simulink library "TLMLib"  (Simulink 8.8)
settings: Solver=VariableStepAuto  StartTime=0.0  StopTime=10.0  RelTol=1e-3
libraries: mblibv1 x12, TLMLib x2
settings Model: Creator=Administrator  LastModifiedBy=robbr48  ExtModeAutoUpdateStatusClock=off

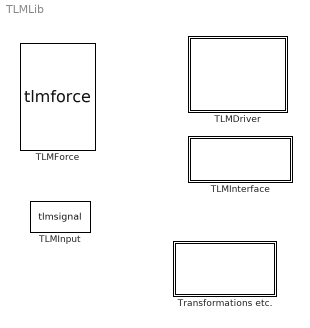
== system TLMLib ==
  TLMDriver : Subsystem
  TLMForce : S-Function  FunctionName=tlmforce  SFunctionDeploymentMode=off  EnableBusSupport=off  mask(TLMForceInterface){}
      mask help:
      | The TLM force interface enables Simulink to participate in TLM Co-Simulations.
      | The interface consists of communication port and a cartesian coordiante system.
      mask Help:
      | The input are:<br>
      | R = Three dimensional position vector, describing the interface location relative the inertial system.<br>
      | A = Orientation matrix 3x3 describing the interface orientation relative the inertial system.<br>
      | vR = Three dimensional velocity vector. <br>
      | Omega = Three dimensional vector describing the rotational velocity.<br>
      | <br>
      | The outputs are:<br>
      | F = Reaction force in the interface.<br>
      | M = Reaction moment in the interface.<br>
      mask Display:
      | port_label('input',1,'R');
      | port_label('input',2,'A');
      | port_label('output',3,'R');
      | port_label('output',4,'A');
      | color('red');
      | port_label('input',3,'vR');
      | port_label('input',4,'Omega');
      | port_label('output',1,'F');
      | port_label('output',2,'M');
  TLMInput : S-Function  FunctionName=tlmsignal  SFunctionDeploymentMode=off  EnableBusSupport=off
      mask Display:
      | port_label('input',1,'u1');
      | port_label('input',2,'u2');
      | color('red');
      | port_label('output',1,'y1');
      | port_label('output',2,'y2');
  TLMInterface : Subsystem
  Transformations etc. : Subsystem
      mask Display: disp('TOOLS')

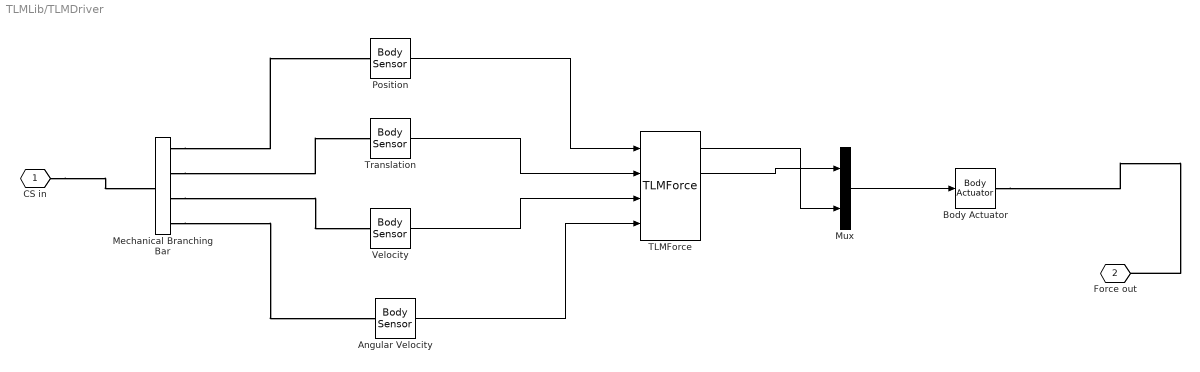
== system TLMLib/TLMDriver ==
  Angular Velocity : mblibv1/Sensors &  Actuators/Body Sensor  SystemSampleTime=-1  PhysicalDomain=Mechanical  PortType=blob  Muxed=on  Pose=off  Angle=on  AngleUnits=deg  ArcVelocity=on  ArcVelocityUnits=rad/s  ArcAcceleration=off  ArcAccelerationUnits=deg/s^2  CoordPosition=off  CoordPositionUnits=m  Velocity=off  VelocityUnits=m/s  Acceleration=off  AccelerationUnits=m/s^2  Quaternion=on  QuaternionDT=off  QuaternionDDT=off  QuaternionUnits=off  OutputVector=[1]  ActiveIO=off  Width=1  DialogClass=MechanicalSensorBlock  ReferenceFrame=Absolute (World)
  Body Actuator : mblibv1/Sensors &  Actuators/Body Actuator  SystemSampleTime=-1  PhysicalDomain=Mechanical  PortType=blob  ActuationStyle=Force  AngleUnits=deg  ArcVelocityUnits=deg/s  ArcAccelerationUnits=deg/s^2  CoordPositionUnits=m  VelocityUnits=m/s  AccelerationUnits=m/s^2  ForceUnits=N  TorqueUnits=N*m  ActiveIO=off  Width=1  DialogClass=MechanicalActuatorBlock  ReferenceFrame=Absolute (World)  Angle=off  CoordPosition=on  Force=on  Torque=on
  Mechanical Branching Bar : mblibv1/Utilities/Mechanical Branching Bar  PhysicalDomain=mechanical  SubClassName=Unknown  LeftPortType=blob  RightPortType=blob  LConnTagsString=_newl0  RConnTagsString=__newr0|SA2|SA3|SA4  DialogClass=MechanicalBranchingBarBlock  NumSAPorts=4
  Mux : Mux  Inputs=[3 3]
  Position : mblibv1/Sensors &  Actuators/Body Sensor  SystemSampleTime=-1  PhysicalDomain=Mechanical  PortType=blob  Muxed=on  Pose=off  Angle=on  AngleUnits=deg  ArcVelocity=off  ArcVelocityUnits=deg/s  ArcAcceleration=off  ArcAccelerationUnits=deg/s^2  CoordPosition=on  CoordPositionUnits=m  Velocity=off  VelocityUnits=m/s  Acceleration=off  AccelerationUnits=m/s^2  Quaternion=on  QuaternionDT=off  QuaternionDDT=off  QuaternionUnits=off  OutputVector=[1]  ActiveIO=off  Width=1  DialogClass=MechanicalSensorBlock  ReferenceFrame=Absolute (World)
  TLMForce : TLMLib/TLMForce
  Translation : mblibv1/Sensors &  Actuators/Body Sensor  SystemSampleTime=-1  PhysicalDomain=Mechanical  PortType=blob  Muxed=on  Pose=on  Angle=on  AngleUnits=deg  ArcVelocity=off  ArcVelocityUnits=deg/s  ArcAcceleration=off  ArcAccelerationUnits=deg/s^2  CoordPosition=off  CoordPositionUnits=m  Velocity=off  VelocityUnits=m/s  Acceleration=off  AccelerationUnits=m/s^2  Quaternion=on  QuaternionDT=off  QuaternionDDT=off  QuaternionUnits=off  OutputVector=[1]  ActiveIO=off  Width=1  DialogClass=MechanicalSensorBlock  ReferenceFrame=Absolute (World)
  Velocity : mblibv1/Sensors &  Actuators/Body Sensor  SystemSampleTime=-1  PhysicalDomain=Mechanical  PortType=blob  Muxed=on  Pose=off  Angle=on  AngleUnits=deg  ArcVelocity=off  ArcVelocityUnits=deg/s  ArcAcceleration=off  ArcAccelerationUnits=deg/s^2  CoordPosition=off  CoordPositionUnits=m  Velocity=on  VelocityUnits=m/s  Acceleration=off  AccelerationUnits=m/s^2  Quaternion=on  QuaternionDT=off  QuaternionDDT=off  QuaternionUnits=off  OutputVector=[1]  ActiveIO=off  Width=1  DialogClass=MechanicalSensorBlock  ReferenceFrame=Absolute (World)
  CS in : PMIOPort  Tag=PMCPort  Port=1  Side=Left
  Force out : PMIOPort  Tag=PMCPort  Port=2  Side=Right
  wires:
  Mux/1 -> Body Actuator/1
  TLMForce/1 -> Mux/2
  TLMForce/2 -> Mux/1
  Angular Velocity/1 -> TLMForce/4
  Velocity/1 -> TLMForce/3
  Translation/1 -> TLMForce/2
  Position/1 -> TLMForce/1
  connections:
  Mechanical Branching Bar/RConn3 -- Velocity/LConn1
  Mechanical Branching Bar/RConn2 -- Translation/LConn1
  Body Actuator/RConn1 -- Force out/RConn1
  CS in/RConn1 -- Mechanical Branching Bar/LConn1
  Mechanical Branching Bar/RConn4 -- Angular Velocity/LConn1
  Mechanical Branching Bar/RConn1 -- Position/LConn1

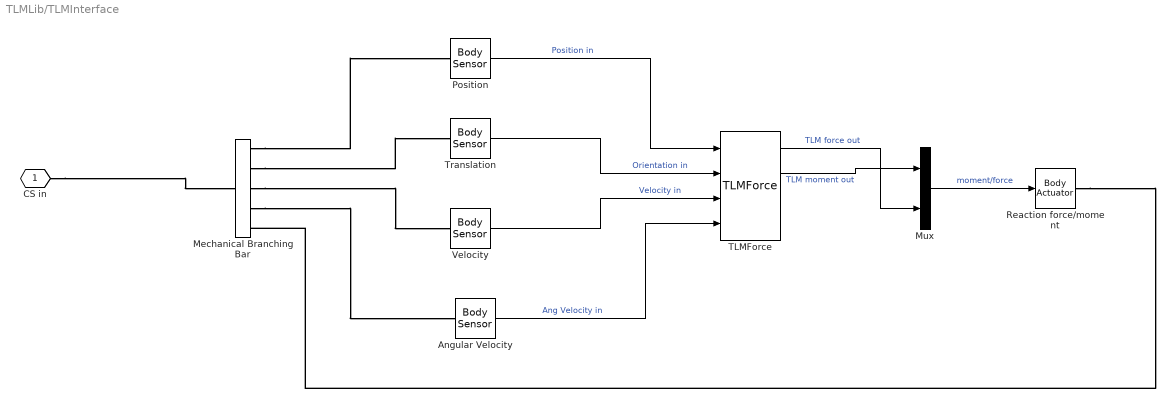
== system TLMLib/TLMInterface ==
  Angular Velocity : mblibv1/Sensors &  Actuators/Body Sensor  SystemSampleTime=-1  PhysicalDomain=Mechanical  PortType=blob  Muxed=on  Pose=off  Angle=on  AngleUnits=deg  ArcVelocity=on  ArcVelocityUnits=rad/s  ArcAcceleration=off  ArcAccelerationUnits=deg/s^2  CoordPosition=off  CoordPositionUnits=m  Velocity=off  VelocityUnits=m/s  Acceleration=off  AccelerationUnits=m/s^2  Quaternion=on  QuaternionDT=off  QuaternionDDT=off  QuaternionUnits=off  OutputVector=[1]  ActiveIO=off  Width=1  DialogClass=MechanicalSensorBlock  ReferenceFrame=Absolute (World)
  Mechanical Branching Bar : mblibv1/Utilities/Mechanical Branching Bar  PhysicalDomain=mechanical  SubClassName=Unknown  LeftPortType=blob  RightPortType=blob  LConnTagsString=_newl0  RConnTagsString=__newr0|SA2|SA3|SA4|SA5  DialogClass=MechanicalBranchingBarBlock  NumSAPorts=5
  Mux : Mux  Inputs=[3 3]
  Position : mblibv1/Sensors &  Actuators/Body Sensor  SystemSampleTime=-1  PhysicalDomain=Mechanical  PortType=blob  Muxed=on  Pose=off  Angle=on  AngleUnits=deg  ArcVelocity=off  ArcVelocityUnits=deg/s  ArcAcceleration=off  ArcAccelerationUnits=deg/s^2  CoordPosition=on  CoordPositionUnits=m  Velocity=off  VelocityUnits=m/s  Acceleration=off  AccelerationUnits=m/s^2  Quaternion=on  QuaternionDT=off  QuaternionDDT=off  QuaternionUnits=off  OutputVector=[1]  ActiveIO=off  Width=1  DialogClass=MechanicalSensorBlock  ReferenceFrame=Absolute (World)
  Reaction force/moment : mblibv1/Sensors &  Actuators/Body Actuator  SystemSampleTime=-1  PhysicalDomain=Mechanical  PortType=blob  ActuationStyle=Force  AngleUnits=deg  ArcVelocityUnits=deg/s  ArcAccelerationUnits=deg/s^2  CoordPositionUnits=m  VelocityUnits=m/s  AccelerationUnits=m/s^2  ForceUnits=N  TorqueUnits=N*m  ActiveIO=off  Width=1  DialogClass=MechanicalActuatorBlock  ReferenceFrame=Absolute (World)  Angle=off  CoordPosition=on  Force=on  Torque=on
  TLMForce : TLMLib/TLMForce
  Translation : mblibv1/Sensors &  Actuators/Body Sensor  SystemSampleTime=-1  PhysicalDomain=Mechanical  PortType=blob  Muxed=on  Pose=on  Angle=on  AngleUnits=deg  ArcVelocity=off  ArcVelocityUnits=deg/s  ArcAcceleration=off  ArcAccelerationUnits=deg/s^2  CoordPosition=off  CoordPositionUnits=m  Velocity=off  VelocityUnits=m/s  Acceleration=off  AccelerationUnits=m/s^2  Quaternion=on  QuaternionDT=off  QuaternionDDT=off  QuaternionUnits=off  OutputVector=[1]  ActiveIO=off  Width=1  DialogClass=MechanicalSensorBlock  ReferenceFrame=Absolute (World)
  Velocity : mblibv1/Sensors &  Actuators/Body Sensor  SystemSampleTime=-1  PhysicalDomain=Mechanical  PortType=blob  Muxed=on  Pose=off  Angle=on  AngleUnits=deg  ArcVelocity=off  ArcVelocityUnits=deg/s  ArcAcceleration=off  ArcAccelerationUnits=deg/s^2  CoordPosition=off  CoordPositionUnits=m  Velocity=on  VelocityUnits=m/s  Acceleration=off  AccelerationUnits=m/s^2  Quaternion=on  QuaternionDT=off  QuaternionDDT=off  QuaternionUnits=off  OutputVector=[1]  ActiveIO=off  Width=1  DialogClass=MechanicalSensorBlock  ReferenceFrame=Absolute (World)
  CS in : PMIOPort  Tag=PMCPort  Port=1  Side=Left
  wires:
  Mux/1 -> Reaction force/moment/1  "moment/force"
  TLMForce/1 -> Mux/2  "TLM force out"
  TLMForce/2 -> Mux/1  "TLM moment out"
  Angular Velocity/1 -> TLMForce/4  "Ang Velocity in"
  Velocity/1 -> TLMForce/3  "Velocity in"
  Translation/1 -> TLMForce/2  "Orientation in"
  Position/1 -> TLMForce/1  "Position in"
  connections:
  Reaction force/moment/RConn1 -- Mechanical Branching Bar/RConn5
  Mechanical Branching Bar/RConn3 -- Velocity/LConn1
  Mechanical Branching Bar/RConn2 -- Translation/LConn1
  CS in/RConn1 -- Mechanical Branching Bar/LConn1
  Mechanical Branching Bar/RConn4 -- Angular Velocity/LConn1
  Mechanical Branching Bar/RConn1 -- Position/LConn1

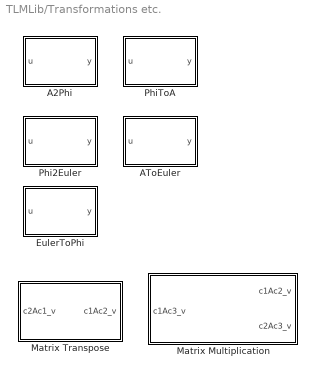
== system TLMLib/Transformations etc. ==
  A2Phi : MATLAB Function  TreatAsAtomicUnit=on
  AToEuler : MATLAB Function  TreatAsAtomicUnit=on
  EulerToPhi : MATLAB Function  TreatAsAtomicUnit=on
  Matrix Multiplication : MATLAB Function  TreatAsAtomicUnit=on
  Matrix Transpose : MATLAB Function  TreatAsAtomicUnit=on
  Phi2Euler : MATLAB Function  TreatAsAtomicUnit=on
  PhiToA : MATLAB Function  TreatAsAtomicUnit=on

== matlab function Transformations etc./A2Phi ==
  data: u input double; y output double
function y = A2Phi321(u)
% This block supports an embeddable subset of the MATLAB language.
% See the help menu for details. 

a11 = u(1);
a12 = u(2);
a13 = u(3);
a23 = u(6);
a33 = u(9);

phi2 = -asin(a13);
cosphi2 = cos(phi2);

phi1 = atan2(a23/cosphi2, a33/cosphi2);
phi3 = atan2(a12/cosphi2, a11/cosphi2);
    
y = [phi1 phi2 phi3];

== matlab function Transformations etc./Phi2Euler ==
  data: u input double; y output double
function y = Phi2E(u)
% This block supports an embeddable subset of the MATLAB language.
% See the help menu for details. 
c1 = cos(u(1)/2.0);
s1 = sin(u(1)/2.0);
c2 = cos(u(2)/2.0);
s2 = sin(u(2)/2.0);
c3 = cos(u(3)/2.0);
s3 = sin(u(3)/2.0);
    
q1 =  s1*c2*c3 - c1*s2*s3 ;
q2 =  c1*s2*c3 + s1*c2*s3 ;
q3 = -s1*s2*c3 + c1*c2*s3 ;
q4 =  c1*c2*c3 + s1*s2*s3 ;

y = [q1 q2 q3 q4];

== matlab function Transformations etc./AToEuler ==
  data: u input double; y output double
function y = A2E(u)
% This block supports an embeddable subset of the MATLAB language.
% See the help menu for details. 

a11 = u(0);
a12 = u(1);
a13 = u(2);
a21 = u(3);
a22 = u(4);
a23 = u(5);
a31 = u(6);
a32 = u(7);
a33 = u(8);

q1 = 0.5*sqrt(Max(0.0,1+a11-a22-a33));
q2 = 0.5*sqrt(Max(0.0,1-a11+a22-a33));
q3 = 0.5*sqrt(Max(0.0,1-a11-a22+a33));
q4 = 0.5*sqrt(Max(0.0,1+a11+a22+a33));
    
if (q1>=q2 && q1>=q3 && q1>=q4) 
	if (a12+a21<0) q2 = -q2; end;
	if (a13+a31<0) q3 = -q3; end;
	if (a23-a32<0) q4 = -q4; end;
elseif (q2>=q1 && q2>=q3 && q2>=q4) 
	if (a12+a21<0) q1 = -q1; end;
	if (a23+a32<0) q3 = -q3; end;
	if (a31-a13<0) q4 = -q4; end;
elseif (q3>=q1 && q3>=q2 && q3>=q4) 
	if (a13+a31<0) q1 = -q1; end;
	if (a23+a32<0) q2 = -q2; end;
	if (a12-a21<0) q4 = -q4; end;
else 
	if (a23-a32<0) q1 = -q1; end;
	if (a31-a13<0) q2 = -q2; end;
	if (a12-a21<0) q3 = -q3; end;
end;

% We choose the solution such that 
% q1 is always positive
if (q1 < 0) 
	q1 = -q1;
	q2 = -q2;
	q3 = -q3;
	q4 = -q4;
end;    


y = [q1 q2 q3 q4];

== matlab function Transformations etc./EulerToPhi ==
  data: u input double; y output double
function y = E2Phi(u)
% This block supports an embeddable subset of the MATLAB language.
% See the help menu for details. 

a11 = u(0)*u(0) - u(1)*u(1) - u(2)*u(2) + u(3)*u(3) ;
a12 = 2.0*(u(0)*u(1) + u(2)*u(3)) ;
a13 = 2.0*(u(0)*u(2) - u(1)*u(3)) ;
a23 = 2.0*(u(1)*u(2) + u(0)*u(3)) ;
a33 = u(2)*u(2) - u(0)*u(0) - u(1)*u(1) + u(3)*u(3) ;

a13 = max(a13, -1);
a13 = min(a13, 1);
phi2 = -asin(a13); % Safe

tmp = cos(phi2) ;
cosphi2 = tmp+Sign(tmp)*1.0e-50 ;
  
% This implementation limits ph1 and phi3 to +/-pi
% so we use it.
phi1 = atan2(a23/cosphi2, a33/cosphi2);
phi3 = atan2(a12/cosphi2, a11/cosphi2);
    

y = [phi1 phi2 phi3];

== matlab function Transformations etc./Matrix Multiplication ==
  data: c1Ac2_v input double; c1Ac3_v output double; c2Ac3_v input double
function c1Ac3_v = MatMult(c1Ac2_v, c2Ac3_v)
% This block supports an embeddable subset of the MATLAB language.
% See the help menu for details. 

% Vector to matrix
c1Ac2=zeros(3,3);
c1Ac2(:)=c1Ac2_v;
c1Ac2=c1Ac2';

% Vector to matrix
c2Ac3=zeros(3,3);
c2Ac3(:)=c2Ac3_v;
c2Ac3=c2Ac3';

% Calc resulting matrix 
c1Ac3=c1Ac2*c2Ac3;
c1Ac3=c1Ac3';

% Return as vector
c1Ac3_v = c1Ac3(:);

== matlab function Transformations etc./Matrix Transpose ==
  data: c1Ac2_v input double; c2Ac1_v output double
function c2Ac1_v = T(c1Ac2_v)
% This block supports an embeddable subset of the MATLAB language.
% See the help menu for details. 

% Vector to matrix
c1Ac2=zeros(3,3);
c1Ac2(:)=c1Ac2_v;

%Transpose
c2Ac1=c1Ac2';

% Return as vector
c2Ac1_v = c2Ac1(:);

== matlab function Transformations etc./PhiToA ==
  data: u input double; y output double
function y = A321(u)
% This block supports an embeddable subset of the MATLAB language.
% See the help menu for details. 

y = [cos(u(2))*cos(u(3)) cos(u(2))*sin(u(3)) -sin(u(2)) -cos(u(1))*sin(u(3))+sin(u(1))*sin(u(2))*cos(u(3)) cos(u(1))*cos(u(3))+sin(u(1))*sin(u(2))*sin(u(3)) sin(u(1))*cos(u(2)) sin(u(1))*sin(u(3))+cos(u(1))*sin(u(2))*cos(u(3)) -sin(u(1))*cos(u(3))+cos(u(1))*sin(u(2))*sin(u(3)) cos(u(1))*cos(u(2))];
